simulink model "PIDautoajustavel"  (R2016b)
settings: Solver=VariableStepAuto  StartTime=0.0  StopTime=120  RelTol=1e-3
undefined symbols (not defined in the file): pulse
libraries: simulink x7
settings Model: Creator=jayme  LastModifiedBy=jayme

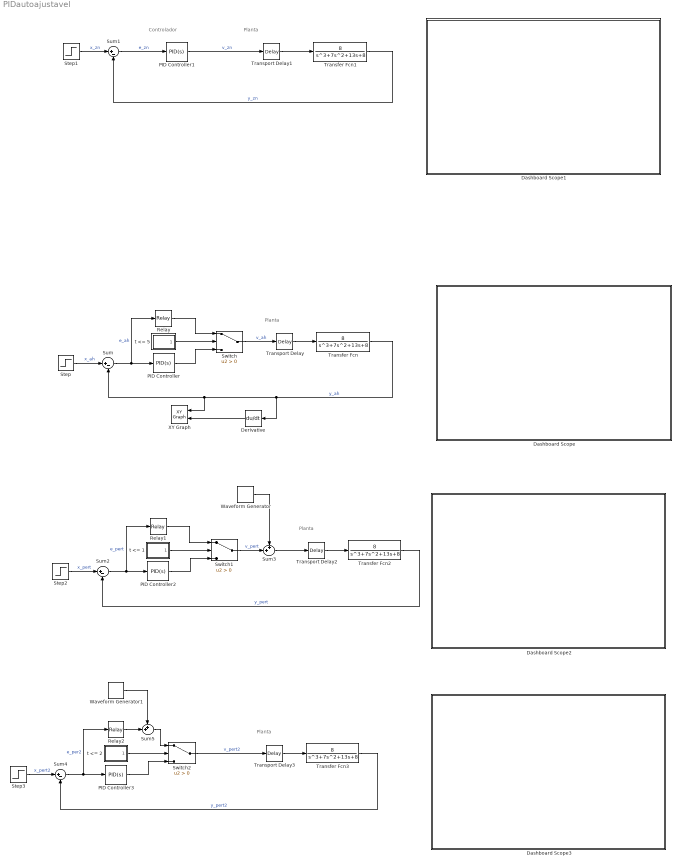
== system PIDautoajustavel ==
  note: Planta
  note: Controlador
  note: Planta
  note: Planta
  note: Planta
  Dashboard Scope : Subsystem  DialogController=hmiCreateDDGDialog  IsWebBlock=on  mask(MWDashboardBlock){webBlockId=38b65158-388b-4ba3-8cb3-0b69bfd1bb03, webBlockType=sdiscope, ShowInitialText=on, HMISrcModelName=PIDautoajustavel}
      mask prompts: webBlockId "WebBlock Id"; webBlockType "WebBlock Type"; HMISrcModelName "Source Model"
      mask help: SimulinkHMI:dialogs:HMIScopeDialogDesc
      mask Help: helpview([docroot '/mapfiles/simulink.map'], 'hmi_scope')
      mask Display:
      | if strcmp(get_param(bdroot(gcb),'BlockDiagramType'), 'library')
      |     image([(matlabroot) '/toolbox/simulink/hmi/icons/DashboardScope.png']);
      | end
  Dashboard Scope1 : Subsystem  DialogController=hmiCreateDDGDialog  IsWebBlock=on  mask(MWDashboardBlock){webBlockId=7bf14781-9dc7-45d6-87ad-77a4c9bf812c, webBlockType=sdiscope, ShowInitialText=on, HMISrcModelName=PIDautoajustavel}
      mask prompts: webBlockId "WebBlock Id"; webBlockType "WebBlock Type"; HMISrcModelName "Source Model"
      mask help: SimulinkHMI:dialogs:HMIScopeDialogDesc
      mask Help: helpview([docroot '/mapfiles/simulink.map'], 'hmi_scope')
      mask Display:
      | if strcmp(get_param(bdroot(gcb),'BlockDiagramType'), 'library')
      |     image([(matlabroot) '/toolbox/simulink/hmi/icons/DashboardScope.png']);
      | end
  Dashboard Scope2 : Subsystem  DialogController=hmiCreateDDGDialog  IsWebBlock=on  mask(MWDashboardBlock){webBlockId=0109d88c-cdcf-418c-b877-ddc8e0d965c3, webBlockType=sdiscope, ShowInitialText=on, HMISrcModelName=PIDautoajustavel}
      mask prompts: webBlockId "WebBlock Id"; webBlockType "WebBlock Type"; HMISrcModelName "Source Model"
      mask help: SimulinkHMI:dialogs:HMIScopeDialogDesc
      mask Help: helpview([docroot '/mapfiles/simulink.map'], 'hmi_scope')
      mask Display:
      | if strcmp(get_param(bdroot(gcb),'BlockDiagramType'), 'library')
      |     image([(matlabroot) '/toolbox/simulink/hmi/icons/DashboardScope.png']);
      | end
  Dashboard Scope3 : Subsystem  DialogController=hmiCreateDDGDialog  IsWebBlock=on  mask(MWDashboardBlock){webBlockId=3226eebf-eb62-4c45-9241-722631610188, webBlockType=sdiscope, ShowInitialText=on, HMISrcModelName=PIDautoajustavel}
      mask prompts: webBlockId "WebBlock Id"; webBlockType "WebBlock Type"; HMISrcModelName "Source Model"
      mask help: SimulinkHMI:dialogs:HMIScopeDialogDesc
      mask Help: helpview([docroot '/mapfiles/simulink.map'], 'hmi_scope')
      mask Display:
      | if strcmp(get_param(bdroot(gcb),'BlockDiagramType'), 'library')
      |     image([(matlabroot) '/toolbox/simulink/hmi/icons/DashboardScope.png']);
      | end
  Derivative : Derivative
  PID Controller : simulink/Continuous/PID Controller  Controller=PID  TimeDomain=Continuous-time  SampleTime=-1  IntegratorMethod=Forward Euler  FilterMethod=Forward Euler  Form=Parallel  UseFilter=on  ControllerParametersSource=internal  P=1.107  I=0.471  D=1.083  N=0.00000001  InitialConditionSource=internal  InitialConditionForIntegrator=0  InitialConditionForFilter=0  ExternalReset=none  LimitOutput=off  UpperSaturationLimit=inf  LowerSaturationLimit=-inf  LinearizeAsGain=on  AntiWindupMode=none  Kb=1  TrackingMode=off  Kt=1  PParamMin=[]  PParamMax=[]  IParamMin=[]  IParamMax=[]  DParamMin=[]  DParamMax=[]  NParamMin=[]  NParamMax=[]  KbParamMin=[]  KbParamMax=[]  KtParamMin=[]  KtParamMax=[]  POutMin=[]  POutMax=[]  IOutMin=[]  IOutMax=[]  DOutMin=[]  DOutMax=[]  NOutMin=[]  NOutMax=[]  KbOutMin=[]  KbOutMax=[]  KtOutMin=[]  KtOutMax=[]  IntegratorOutMin=[]  IntegratorOutMax=[]  FilterOutMin=[]  FilterOutMax=[]  SumOutMin=[]  SumOutMax=[]  SumI1OutMin=[]  SumI1OutMax=[]  SumI2OutMin=[]  SumI2OutMax=[]  SumI3OutMin=[]  SumI3OutMax=[]  SumDOutMin=[]  SumDOutMax=[]  SaturationOutMin=[]  SaturationOutMax=[]  IntegratorContinuousStateAttributes=''  IntegratorStateMustResolveToSignalObject=off  IntegratorRTWStateStorageClass=Auto  FilterContinuousStateAttributes=''  FilterStateMustResolveToSignalObject=off  FilterRTWStateStorageClass=Auto  DifferentiatorICPrevScaledInput=0  DifferentiatorOutMin=[]  DifferentiatorOutMax=[]
  PID Controller1 : simulink/Continuous/PID Controller  Controller=PID  TimeDomain=Continuous-time  SampleTime=-1  IntegratorMethod=Forward Euler  FilterMethod=Forward Euler  Form=Parallel  UseFilter=on  ControllerParametersSource=internal  P=1.14  I=0.465  D=1.159  N=0.0000001  InitialConditionSource=internal  InitialConditionForIntegrator=0  InitialConditionForFilter=0  ExternalReset=none  LimitOutput=off  UpperSaturationLimit=inf  LowerSaturationLimit=-inf  LinearizeAsGain=on  AntiWindupMode=none  Kb=1  TrackingMode=off  Kt=1  PParamMin=[]  PParamMax=[]  IParamMin=[]  IParamMax=[]  DParamMin=[]  DParamMax=[]  NParamMin=[]  NParamMax=[]  KbParamMin=[]  KbParamMax=[]  KtParamMin=[]  KtParamMax=[]  POutMin=[]  POutMax=[]  IOutMin=[]  IOutMax=[]  DOutMin=[]  DOutMax=[]  NOutMin=[]  NOutMax=[]  KbOutMin=[]  KbOutMax=[]  KtOutMin=[]  KtOutMax=[]  IntegratorOutMin=[]  IntegratorOutMax=[]  FilterOutMin=[]  FilterOutMax=[]  SumOutMin=[]  SumOutMax=[]  SumI1OutMin=[]  SumI1OutMax=[]  SumI2OutMin=[]  SumI2OutMax=[]  SumI3OutMin=[]  SumI3OutMax=[]  SumDOutMin=[]  SumDOutMax=[]  SaturationOutMin=[]  SaturationOutMax=[]  IntegratorContinuousStateAttributes=''  IntegratorStateMustResolveToSignalObject=off  IntegratorRTWStateStorageClass=Auto  FilterContinuousStateAttributes=''  FilterStateMustResolveToSignalObject=off  FilterRTWStateStorageClass=Auto  DifferentiatorICPrevScaledInput=0  DifferentiatorOutMin=[]  DifferentiatorOutMax=[]
  PID Controller2 : simulink/Continuous/PID Controller  Controller=PID  TimeDomain=Continuous-time  SampleTime=-1  IntegratorMethod=Forward Euler  FilterMethod=Forward Euler  Form=Parallel  UseFilter=on  ControllerParametersSource=internal  P=1.107  I=0.471  D=1.083  N=0.00000001  InitialConditionSource=internal  InitialConditionForIntegrator=0  InitialConditionForFilter=0  ExternalReset=none  LimitOutput=off  UpperSaturationLimit=inf  LowerSaturationLimit=-inf  LinearizeAsGain=on  AntiWindupMode=none  Kb=1  TrackingMode=off  Kt=1  PParamMin=[]  PParamMax=[]  IParamMin=[]  IParamMax=[]  DParamMin=[]  DParamMax=[]  NParamMin=[]  NParamMax=[]  KbParamMin=[]  KbParamMax=[]  KtParamMin=[]  KtParamMax=[]  POutMin=[]  POutMax=[]  IOutMin=[]  IOutMax=[]  DOutMin=[]  DOutMax=[]  NOutMin=[]  NOutMax=[]  KbOutMin=[]  KbOutMax=[]  KtOutMin=[]  KtOutMax=[]  IntegratorOutMin=[]  IntegratorOutMax=[]  FilterOutMin=[]  FilterOutMax=[]  SumOutMin=[]  SumOutMax=[]  SumI1OutMin=[]  SumI1OutMax=[]  SumI2OutMin=[]  SumI2OutMax=[]  SumI3OutMin=[]  SumI3OutMax=[]  SumDOutMin=[]  SumDOutMax=[]  SaturationOutMin=[]  SaturationOutMax=[]  IntegratorContinuousStateAttributes=''  IntegratorStateMustResolveToSignalObject=off  IntegratorRTWStateStorageClass=Auto  FilterContinuousStateAttributes=''  FilterStateMustResolveToSignalObject=off  FilterRTWStateStorageClass=Auto  DifferentiatorICPrevScaledInput=0  DifferentiatorOutMin=[]  DifferentiatorOutMax=[]
  PID Controller3 : simulink/Continuous/PID Controller  Controller=PID  TimeDomain=Continuous-time  SampleTime=-1  IntegratorMethod=Forward Euler  FilterMethod=Forward Euler  Form=Parallel  UseFilter=on  ControllerParametersSource=internal  P=1.107  I=0.471  D=1.083  N=0.00000001  InitialConditionSource=internal  InitialConditionForIntegrator=0  InitialConditionForFilter=0  ExternalReset=none  LimitOutput=off  UpperSaturationLimit=inf  LowerSaturationLimit=-inf  LinearizeAsGain=on  AntiWindupMode=none  Kb=1  TrackingMode=off  Kt=1  PParamMin=[]  PParamMax=[]  IParamMin=[]  IParamMax=[]  DParamMin=[]  DParamMax=[]  NParamMin=[]  NParamMax=[]  KbParamMin=[]  KbParamMax=[]  KtParamMin=[]  KtParamMax=[]  POutMin=[]  POutMax=[]  IOutMin=[]  IOutMax=[]  DOutMin=[]  DOutMax=[]  NOutMin=[]  NOutMax=[]  KbOutMin=[]  KbOutMax=[]  KtOutMin=[]  KtOutMax=[]  IntegratorOutMin=[]  IntegratorOutMax=[]  FilterOutMin=[]  FilterOutMax=[]  SumOutMin=[]  SumOutMax=[]  SumI1OutMin=[]  SumI1OutMax=[]  SumI2OutMin=[]  SumI2OutMax=[]  SumI3OutMin=[]  SumI3OutMax=[]  SumDOutMin=[]  SumDOutMax=[]  SaturationOutMin=[]  SaturationOutMax=[]  IntegratorContinuousStateAttributes=''  IntegratorStateMustResolveToSignalObject=off  IntegratorRTWStateStorageClass=Auto  FilterContinuousStateAttributes=''  FilterStateMustResolveToSignalObject=off  FilterRTWStateStorageClass=Auto  DifferentiatorICPrevScaledInput=0  DifferentiatorOutMin=[]  DifferentiatorOutMax=[]
  Relay : Relay  OnSwitchValue=0  OffSwitchValue=0  OffOutputValue=-1
  Relay1 : Relay  OnSwitchValue=0  OffSwitchValue=0  OffOutputValue=-1
  Relay2 : Relay  OnSwitchValue=0  OffSwitchValue=0  OffOutputValue=-1
  Step{,1..3} (4 alike) : Step  Time=80  SampleTime=0
  Sum{,1..2,4} (4 alike) : Sum  Inputs=|+-
  Sum3 : Sum  Inputs=++|
  Sum5 : Sum  Inputs=++|
  Switch : Switch  Criteria=u2 > Threshold
  Switch1 : Switch  Criteria=u2 > Threshold
  Switch2 : Switch  Criteria=u2 > Threshold
  Transfer Fcn{,1..3} (4 alike) : TransferFcn  Numerator=[8]  Denominator=[1 7 13 8]
  Transport Delay{,1..3} (4 alike) : TransportDelay
  Waveform Generator : simulink/Sources/Waveform Generator  OutMin=[]  OutMax=[]  OutDataTypeStr=double  SelectedSignal=1  Signals=pulse('Amplitude',1,'TriggerTime',30,'Duration',2)  BlockNames=MultiportSwitch_c9fa51b22c534c8  SampleTime=0.1
  Waveform Generator1 : simulink/Sources/Waveform Generator  OutMin=[]  OutMax=[]  OutDataTypeStr=double  SelectedSignal=1  Signals=gaussian('Mean',0,'Variance',5,'Seed',1)#  BlockNames=MultiportSwitch_7c7d636642ed46e#MultiportSwitch_15035ff7117c4d3  SampleTime=0.1
  XY Graph : simulink/Sinks/XY Graph  xmin=-1  xmax=2  ymin=-1.5  ymax=1.5  st=-1
  t <= 1 : Subsystem
  t <= 2 : Subsystem
  t <= 5 : Subsystem
  wires:
  Step/1 -> Sum/1  "x_ah"
  Sum/1 -> PID Controller/1, Relay/1  "e_ah"
  Transfer Fcn/1 -> Derivative/1, XY Graph/1, Sum/2  "y_ah"
  Transport Delay/1 -> Transfer Fcn/1
  Switch/1 -> Transport Delay/1  "v_ah"
  PID Controller/1 -> Switch/3
  t <= 5/1(t <= 40) -> Switch/2
  Relay/1 -> Switch/1
  Step1/1 -> Sum1/1  "x_zn"
  Sum1/1 -> PID Controller1/1  "e_zn"
  Transfer Fcn1/1 -> Sum1/2  "y_zn"
  Transport Delay1/1 -> Transfer Fcn1/1
  PID Controller1/1 -> Transport Delay1/1  "v_zn"
  Step2/1 -> Sum2/1  "x_pert"
  Sum2/1 -> PID Controller2/1, Relay1/1  "e_pert"
  Transfer Fcn2/1 -> Sum2/2  "y_pert"
  Transport Delay2/1 -> Transfer Fcn2/1
  PID Controller2/1 -> Switch1/3
  t <= 1/1(t <= 20) -> Switch1/2
  Relay1/1 -> Switch1/1
  Switch1/1 -> Sum3/2  "v_pert"
  Sum3/1 -> Transport Delay2/1
  Waveform Generator/1 -> Sum3/1
  Derivative/1 -> XY Graph/2
  Step3/1 -> Sum4/1  "x_pert2"
  Sum4/1 -> PID Controller3/1, Relay2/1  "e_per2"
  Transfer Fcn3/1 -> Sum4/2  "y_pert2"
  Transport Delay3/1 -> Transfer Fcn3/1
  PID Controller3/1 -> Switch2/3
  t <= 2/1(t <= 20) -> Switch2/2
  Relay2/1 -> Sum5/2
  Sum5/1 -> Switch2/1
  Waveform Generator1/1 -> Sum5/1
  Switch2/1 -> Transport Delay3/1  "v_pert2"

== system PIDautoajustavel/Dashboard Scope ==

== system PIDautoajustavel/Dashboard Scope1 ==

== system PIDautoajustavel/Dashboard Scope2 ==

== system PIDautoajustavel/Dashboard Scope3 ==

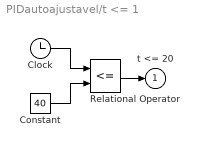
== system PIDautoajustavel/t <= 1 ==
  Clock : Clock
  Constant : Constant  Value=40
  Relational Operator : RelationalOperator  Operator=<=  RndMeth=Nearest  InputSameDT=on
  t <= 20 : Outport  InitialOutput=0
  wires:
  Constant/1 -> Relational Operator/2
  Clock/1 -> Relational Operator/1
  Relational Operator/1 -> t <= 20/1

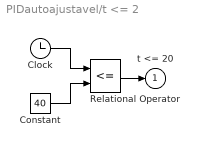
== system PIDautoajustavel/t <= 2 ==
  Clock : Clock
  Constant : Constant  Value=40
  Relational Operator : RelationalOperator  Operator=<=  RndMeth=Nearest  InputSameDT=on
  t <= 20 : Outport  InitialOutput=0
  wires:
  Constant/1 -> Relational Operator/2
  Clock/1 -> Relational Operator/1
  Relational Operator/1 -> t <= 20/1

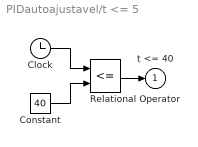
== system PIDautoajustavel/t <= 5 ==
  Clock : Clock
  Constant : Constant  Value=40
  Relational Operator : RelationalOperator  Operator=<=  RndMeth=Nearest  InputSameDT=on
  t <= 40 : Outport  InitialOutput=0
  wires:
  Constant/1 -> Relational Operator/2
  Clock/1 -> Relational Operator/1
  Relational Operator/1 -> t <= 40/1
